simulink model "error_model"  (R2021a)
settings: Solver=VariableStepAuto  StartTime=0.0  StopTime=10.0  RelTol=1e-3
settings Model: Creator=dhruv  LastModifiedBy=dhruv

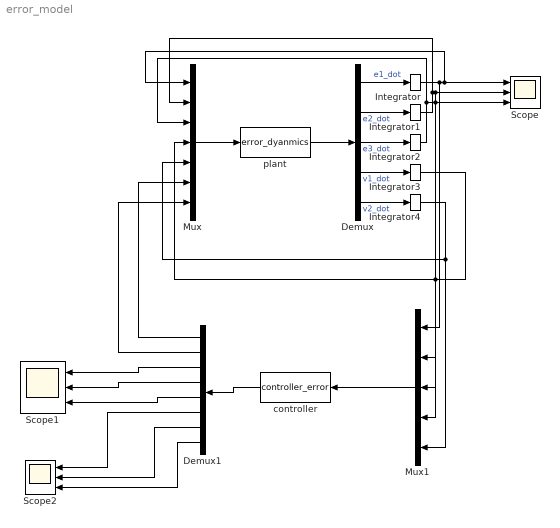
== system error_model ==
  Demux : Demux  Outputs=5
  Demux1 : Demux  Outputs=8
  Integrator : Integrator  InitialCondition=5
  Integrator1 : Integrator  InitialCondition=5
  Integrator2 : Integrator  InitialCondition=3
  Integrator3 : Integrator
  Integrator4 : Integrator
  Mux : Mux  Inputs=7
  Mux1 : Mux  Inputs=5
  Scope : Scope  NumInputPorts=3
  Scope1 : Scope  NumInputPorts=3
  Scope2 : Scope  NumInputPorts=3
  controller : MATLABFcn  MATLABFcn=controller_error  OutputDimensions=8
  plant : MATLABFcn  MATLABFcn=error_dyanmics  OutputDimensions=5
  wires:
  Mux/1 -> plant/1
  plant/1 -> Demux/1
  Demux/1 -> Integrator/1  "e1_dot"
  Demux/2 -> Integrator1/1  "e2_dot"
  Demux/3 -> Integrator2/1  "e3_dot"
  Demux/4 -> Integrator3/1  "v1_dot"
  Demux/5 -> Integrator4/1  "v2_dot"
  Integrator/1 -> Scope/1, Mux/1, Mux1/1
  Integrator1/1 -> Mux1/2, Scope/2, Mux/2
  Integrator2/1 -> Mux1/3, Scope/3, Mux/3
  Integrator3/1 -> Mux1/4, Mux/4
  Integrator4/1 -> Mux1/5, Mux/5
  Mux1/1 -> controller/1
  controller/1 -> Demux1/1
  Demux1/1 -> Mux/6
  Demux1/2 -> Mux/7
  Demux1/3 -> Scope1/1
  Demux1/4 -> Scope1/2
  Demux1/5 -> Scope1/3
  Demux1/6 -> Scope2/1
  Demux1/7 -> Scope2/2
  Demux1/8 -> Scope2/3
